simulink model "gm_commhdlQPSKTxRx"  (R2025b)
settings: Solver=VariableStepAuto  StartTime=0.0  StopTime=10.0  RelTol=1e-3
PostLoadFcn:
  | hScopeConfig = get_param([gcs '/Receiver/QPSK Rx/Frequency and Time Synchronizer/Symbol Synchronizer/No HDL/QPSK Receiver Eye Diagram'],'ScopeConfiguration');
  | 
  | hScopeConfig.OpenAtSimulationStart = false;
  | hScopeConfig.Visible = false;
  | SamplesPerSymbol = 4;
  | %UpsamplesRx = 1;
  | clear hScopeConfig
InitFcn:
  | commhdlQPSKTxRxModelInit;
  | % Rate bridge: ADRV9002/Jupiter radio runs at 15.36 MHz = 2x the 7.68 MHz
  | % (4 samples/symbol @ Rsym=1.92 MHz) the QPSK Rx requires. The deployed
  | % Receiver must downsample the ADC stream by 2. UpsamplesRx=1 fed the QPSK
  | % Rx 8 sps (2x-upsampled) and broke symbol sync / the loopback bit check.
  | UpsamplesRx = 2;
  | UpsamplesTx = 1;
  | clear simTimingOffset;
StopFcn:
  | if exist('simTimingOffset','var')
  |   disp('Simulation completed');
  |   %QPSKTxRxVerification;
  | end
undefined symbols (not defined in the file or in its folder): Add, Config, Error, fsym, Ignore, randsrc, RandStream, Rsym, Shift
libraries: hdlsllib x64, dspsigops x19, simulink x19, dsphdlfiltering2 x3, dsphdlsigops2 x2, dsphdlmathfun2 x2, commdigbbndpm3 x2, commchan3 x1, commrflib2 x1
(part 2 of 9)

== system gm_commhdlQPSKTxRx/Transmitter/QPSK Tx/HDL Data Scrambler ==
  note: HDL Data Scrambler
      | Polynomial: x^7+x^4+1
      | Initial state: [1 0 1 1 1 0 1]
  dataIn : Inport
  startIn : Inport  Port=2
  endIn : Inport  Port=3
  validIn : Inport  Port=4
  BIT_XOR : Logic  Operator=XOR  IconShape=distinctive  AllPortsSameDT=off  OutDataTypeStr=boolean
  BIT_XOR2 : Logic  Operator=XOR  IconShape=distinctive  AllPortsSameDT=off  OutDataTypeStr=boolean
  Delay{,1,3..4} (4 alike) : Delay  DelayLength=1
  EnableScrambling : Constant  Value=true  SampleTime=-1
  Logical Operator : Logic  IconShape=distinctive  AllPortsSameDT=off  OutDataTypeStr=boolean
  Switch : Switch  Criteria=u2 > Threshold  SaturateOnIntegerOverflow=off  InputSameDT=off
  Unit Delay Enabled Resettable Synchronous{,2..3,5,7} (5 alike) : hdlsllib/Discrete/Unit Delay Enabled Resettable Synchronous  InitialCondition=1  SampleTime=-1
  Unit Delay Enabled Resettable Synchronous1 : hdlsllib/Discrete/Unit Delay Enabled Resettable Synchronous  InitialCondition=0  SampleTime=-1
  Unit Delay Enabled Resettable Synchronous4 : hdlsllib/Discrete/Unit Delay Enabled Resettable Synchronous  InitialCondition=0  SampleTime=-1
  Unit Delay Enabled Resettable Synchronous6 : hdlsllib/Discrete/Unit Delay Enabled Resettable Synchronous  InitialCondition=0.0  SampleTime=-1
  dataOut : Outport  InitialOutput=0
  validOut : Outport  Port=2  InitialOutput=0
  wires:
  BIT_XOR2/1 -> Switch/1
  EnableScrambling/1 -> Switch/2
  Switch/1 -> Delay3/1
  Unit Delay Enabled Resettable Synchronous7/1 -> BIT_XOR/1
  Unit Delay Enabled Resettable Synchronous6/1 -> Unit Delay Enabled Resettable Synchronous7/1
  Unit Delay Enabled Resettable Synchronous5/1 -> Unit Delay Enabled Resettable Synchronous6/1
  Unit Delay Enabled Resettable Synchronous3/1 -> Unit Delay Enabled Resettable Synchronous5/1, BIT_XOR/2
  Unit Delay Enabled Resettable Synchronous/1 -> Unit Delay Enabled Resettable Synchronous1/1
  Unit Delay Enabled Resettable Synchronous2/1 -> Unit Delay Enabled Resettable Synchronous3/1
  Unit Delay Enabled Resettable Synchronous1/1 -> Unit Delay Enabled Resettable Synchronous2/1
  BIT_XOR/1 -> Logical Operator/2, Unit Delay Enabled Resettable Synchronous/1
  validIn/1 -> Delay1/1
  dataIn/1 -> Delay/1
  startIn/1 -> Unit Delay Enabled Resettable Synchronous7/3, Unit Delay Enabled Resettable Synchronous3/3, Unit Delay Enabled Resettable Synchronous2/3, Unit Delay Enabled Resettable Synchronous/3, Unit Delay Enabled Resettable Synchronous1/3, Unit Delay Enabled Resettable Synchronous5/3, Unit Delay Enabled Resettable Synchronous6/3, Unit Delay Enabled Resettable Synchronous4/2, Unit Delay Enabled Resettable Synchronous4/1
  Delay/1 -> BIT_XOR2/1, Switch/3
  Delay1/1 -> Unit Delay Enabled Resettable Synchronous7/2, Unit Delay Enabled Resettable Synchronous5/2, Unit Delay Enabled Resettable Synchronous3/2, Delay4/1, Unit Delay Enabled Resettable Synchronous/2, Unit Delay Enabled Resettable Synchronous1/2, Unit Delay Enabled Resettable Synchronous2/2, Unit Delay Enabled Resettable Synchronous6/2
  Unit Delay Enabled Resettable Synchronous4/1 -> Logical Operator/1
  Logical Operator/1 -> BIT_XOR2/2
  endIn/1 -> Unit Delay Enabled Resettable Synchronous4/3
  Delay3/1 -> dataOut/1
  Delay4/1 -> validOut/1

== system gm_commhdlQPSKTxRx/Transmitter/QPSK Tx/QPSK Modulator ==
  dataIn : Inport
  validIn : Inport  Port=2
  Compare To Constant : simulink/Logic and Bit Operations/Compare To Constant  relop===  const=0  OutDataTypeStr=boolean
  Compare To Constant1 : simulink/Logic and Bit Operations/Compare To Constant  relop===  const=1  OutDataTypeStr=boolean
  Delay{,1..5,11..12} (8 alike) : Delay  DelayLength=1
  HDL Counter : hdlsllib/Sources/HDL Counter  CountType=Count limited  CountInit=0  CountStep=1  CountMax=1  CountFromType=Initial value  CountFrom=0  CountResetPort=off  CountLoadPort=off  CountEnbPort=on  CountDirPort=off  CountHitOutputPort=off  CountDataType=Unsigned  CountWordLen=1  CountFracLen=0  CountSampTime=1
  Logical Operator : Logic  IconShape=distinctive  AllPortsSameDT=off  OutDataTypeStr=boolean
  Logical Operator1 : Logic  IconShape=distinctive  AllPortsSameDT=off  OutDataTypeStr=boolean
  Mux : Mux  Inputs=2
  Null : Constant  Value=complex(0,0)  OutDataTypeStr=fixdt(1,16,15)  SampleTime=1/(Rsym*4)
  QPSK Modulator Baseband : commdigbbndpm3/QPSK Modulator Baseband  InType=Bit  Enc=Gray  Ph=pi/4  outDtype=Fixed-point  outWordLen=16  outUDDataType=sfix(16)  outFracLenMode=User-defined  outFracLen=15  outDataTypeStr=fixdt(1,16,15)  outLastDataTypeStr=fixdt(1,16,15)
  Switch3 : Switch  Threshold=1  SaturateOnIntegerOverflow=off  InputSameDT=off
  Unit Delay Enabled Synchronous : hdlsllib/Discrete/Unit Delay Enabled Synchronous  InitialCondition=0.0  SampleTime=-1
  dataOut : Outport
  validOut : Outport  Port=2
  wires:
  Delay5/1 -> Delay12/1
  Delay4/1 -> QPSK Modulator Baseband/1
  Mux/1 -> Delay4/1
  Unit Delay Enabled Synchronous/1 -> Mux/1
  Logical Operator/1 -> Unit Delay Enabled Synchronous/2
  Delay12/1 -> Delay3/1, Switch3/2
  Delay11/1 -> Switch3/1
  Compare To Constant1/1 -> Logical Operator1/1
  Compare To Constant/1 -> Logical Operator/2
  Delay1/1 -> HDL Counter/1, Logical Operator/1, Logical Operator1/2
  Delay3/1 -> validOut/1
  Delay2/1 -> dataOut/1
  Delay/1 -> Unit Delay Enabled Synchronous/1, Mux/2
  Null/1 -> Switch3/3
  Switch3/1 -> Delay2/1
  Logical Operator1/1 -> Delay5/1
  QPSK Modulator Baseband/1 -> Delay11/1
  HDL Counter/1 -> Compare To Constant1/1, Compare To Constant/1
  validIn/1 -> Delay1/1
  dataIn/1 -> Delay/1

== system gm_commhdlQPSKTxRx/Transmitter/QPSK Tx/RRC Transmit Filter ==
  dataIn : Inport
  validIn : Inport  Port=2
  Data Type Conversion : DataTypeConversion  OutDataTypeStr=fixdt(1,17,16)  SaturateOnIntegerOverflow=off  RndMeth=Floor
  Data Type Conversion1 : DataTypeConversion  OutDataTypeStr=fixdt(1,16,14)  SaturateOnIntegerOverflow=off  RndMeth=Floor
  Delay1 : Delay  DelayLength=1
  Delay2 : Delay  DelayLength=1
  Delay3 : Delay  DelayLength=1
  RRC Filter : dsphdlfiltering2/Discrete FIR Filter  NumeratorSource=Property  Numerator=RRCCoef  NumeratorPrototype=[]  FilterStructure=Direct form systolic  SerializationOption=Minimum number of cycles between valid input samples  NumCycles=2  NumberOfMultipliers=2  SimulateUsing=Code generation  roundingMode=Floor  overflowMode=off  CoefficientsDataTypeStr=Inherit: Same word length as input  OutputDataTypeStr=Inherit: Same word length as input  ResetInputPort=off  HDLGlobalReset=off  CoeffMultiplier=Multiplier  UseMultForPow2Coeff=on  FrameInputSymmOptim=off
  Unit Delay Enabled Synchronous1 : hdlsllib/Discrete/Unit Delay Enabled Synchronous  InitialCondition=0  SampleTime=-1
  dataOut : Outport
  validOut : Outport  Port=2
  wires:
  Delay3/1 -> RRC Filter/1
  validIn/1 -> Unit Delay Enabled Synchronous1/1, Unit Delay Enabled Synchronous1/2
  Data Type Conversion1/1 -> Delay1/1
  Unit Delay Enabled Synchronous1/1 -> RRC Filter/2
  Data Type Conversion/1 -> Delay3/1
  Delay2/1 -> validOut/1
  Delay1/1 -> dataOut/1
  RRC Filter/2 -> Delay2/1
  RRC Filter/1 -> Data Type Conversion1/1
  dataIn/1 -> Data Type Conversion/1

== system gm_commhdlQPSKTxRx/Receiver/QPSK Rx/Automatic Gain Control/Error Detector ==
  dataIn : Inport  OutDataTypeStr=fixdt(1, 16, 14)  PortDimensions=1  SampleTime=1.30208333333333e-07
      settings: SignalType=complex
  Add1 : Sum  Inputs=+-  OutDataTypeStr=fixdt(1, 33, 28)
  Conj : Math  Operator=conj  OutDataTypeStr=fixdt(1, 16, 14)
  Delay{,1..3} (4 alike) : Delay
  Product : Product  OutDataTypeStr=fixdt(1, 32, 28)
  Ref : Constant  Value=Ref  OutDataTypeStr=fixdt(1, 16, 14)  SampleTime=-1
  err : Outport  SampleTime=1.30208333333333e-07
  wires:
  Delay3/1 -> err/1
  Add1/1 -> Delay3/1
  Delay2/1 -> Add1/2
  Ref/1 -> Add1/1
  Product/1 -> Delay2/1
  Delay/1 -> Product/2
  Delay1/1 -> Product/1
  Conj/1 -> Delay/1
  dataIn/1 -> Conj/1, Delay1/1

== system gm_commhdlQPSKTxRx/Receiver/QPSK Rx/Automatic Gain Control/Loop Filter ==
  err : Inport  OutDataTypeStr=fixdt(1, 33, 28)  PortDimensions=1  SampleTime=1.30208333333333e-07
      settings: SignalType=complex
  Add : Sum  Inputs=|++  OutDataTypeStr=fixdt(1, 33, 28)
  Delay1 : Delay  DelayLength=1
  Delay2 : Delay
  Delay3 : Delay
  Gain1 : Gain  Gain=LFG  OutDataTypeStr=fixdt(1, 33, 28)
      mask init:
      | Simulink.suppressDiagnostic(gcb, 'SimulinkFixedPoint:util:fxpParameterPrecisionLoss');
  gain : Outport  SampleTime=1.30208333333333e-07
  wires:
  Delay2/1 -> Add/1
  Add/1 -> Delay1/1
  Gain1/1 -> Delay2/1
  Delay3/1 -> Gain1/1
  Delay1/1 -> gain/1, Add/2
  err/1 -> Delay3/1

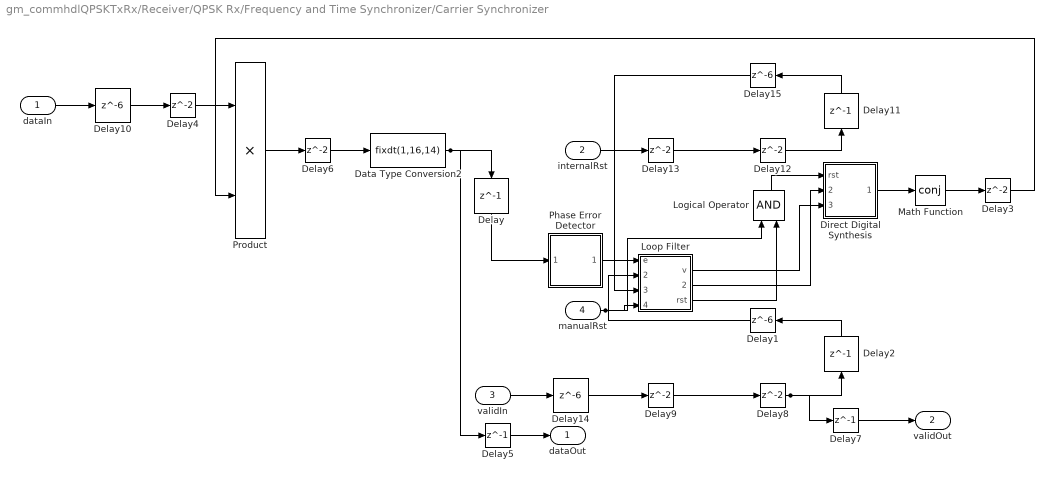
== system gm_commhdlQPSKTxRx/Receiver/QPSK Rx/Frequency and Time Synchronizer/Carrier Synchronizer ==
  dataIn : Inport  OutDataTypeStr=fixdt(1, 16, 14)  PortDimensions=1  SampleTime=1.30208333333333e-07
      settings: SignalType=complex
  internalRst : Inport  Port=2  OutDataTypeStr=boolean  PortDimensions=1  SampleTime=1.30208333333333e-07
  validIn : Inport  Port=3  OutDataTypeStr=boolean  PortDimensions=1  SampleTime=1.30208333333333e-07
  manualRst : Inport  Port=4  OutDataTypeStr=boolean  PortDimensions=1  SampleTime=1.30208333333333e-07
  Data Type Conversion2 : DataTypeConversion  OutDataTypeStr=fixdt(1,16,14)  SaturateOnIntegerOverflow=off  RndMeth=Floor
  Delay{,2,5,7,11} (5 alike) : Delay  DelayLength=1
  Delay{1,10,14..15} (4 alike) : Delay  DelayLength=6
  Delay{3..4,6,8..9,12..13} (7 alike) : Delay
  Direct Digital Synthesis : Subsystem
  Logical Operator : Logic  AllPortsSameDT=off  OutDataTypeStr=boolean
  Loop Filter : Subsystem
  Math Function : Math  Operator=conj  SignedPower=on  OutDataTypeStr=fixdt(1, 16, 14)  RndMeth=Zero
  Phase Error Detector : Subsystem
  Product : Product  OutDataTypeStr=fixdt(1, 32, 28)
  dataOut : Outport  SampleTime=1.30208333333333e-07
  validOut : Outport  Port=2  SampleTime=1.30208333333333e-07
  wires:
  Delay7/1 -> validOut/1
  Delay2/1 -> Delay1/1
  Logical Operator/1 -> Direct Digital Synthesis/1(rst)
  Direct Digital Synthesis/1(expOut) -> Math Function/1
  Delay1/1 -> Loop Filter/2(validIn)
  Loop Filter/3(rst) -> Logical Operator/2
  Delay9/1 -> Delay8/1
  Loop Filter/2(valid) -> Direct Digital Synthesis/2(validIn)
  Loop Filter/1(v) -> Direct Digital Synthesis/3(phaseInc)
  Math Function/1 -> Delay3/1
  Delay12/1 -> Delay11/1
  Delay13/1 -> Delay12/1
  Delay10/1 -> Delay4/1
  Delay3/1 -> Product/2
  Delay11/1 -> Delay15/1
  Data Type Conversion2/1 -> Delay5/1, Delay/1
  internalRst/1 -> Delay13/1
  Product/1 -> Delay6/1
  Delay5/1 -> dataOut/1
  Delay6/1 -> Data Type Conversion2/1
  Delay15/1 -> Loop Filter/3(internalRst)
  manualRst/1 -> Loop Filter/4(externalRst), Logical Operator/1
  Delay4/1 -> Product/1
  Delay14/1 -> Delay9/1
  Delay/1 -> Phase Error Detector/1(dataIn)
  Delay8/1 -> Delay7/1, Delay2/1
  dataIn/1 -> Delay10/1
  validIn/1 -> Delay14/1
  Phase Error Detector/1(PhaseError) -> Loop Filter/1(e)

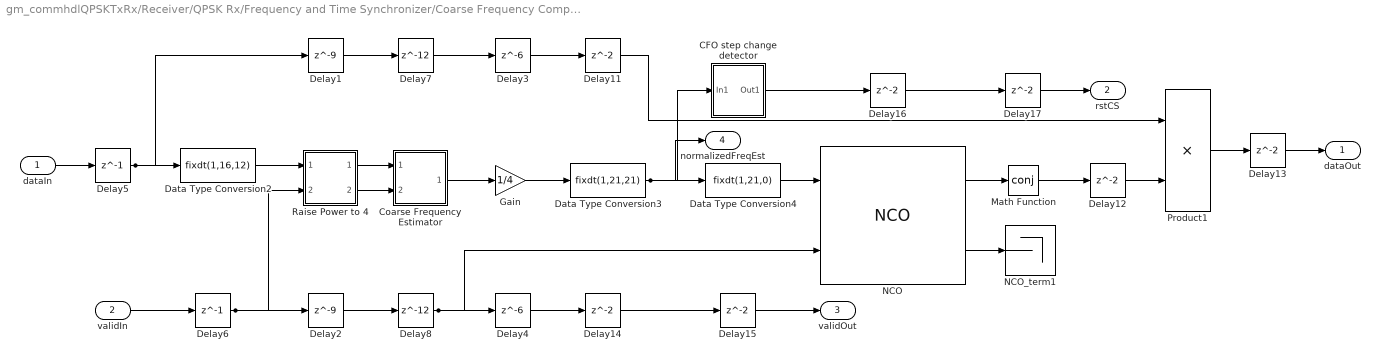
== system gm_commhdlQPSKTxRx/Receiver/QPSK Rx/Frequency and Time Synchronizer/Coarse Frequency Compensator ==
  dataIn : Inport  OutDataTypeStr=fixdt(1, 16, 14)  PortDimensions=1  SampleTime=1.30208333333333e-07
      settings: SignalType=complex
  validIn : Inport  Port=2  OutDataTypeStr=boolean  PortDimensions=1  SampleTime=1.30208333333333e-07
  CFO step change detector : Subsystem
  Coarse Frequency Estimator : Subsystem
  Data Type Conversion2 : DataTypeConversion  OutDataTypeStr=fixdt(1,16,12)  SaturateOnIntegerOverflow=off  RndMeth=Floor
  Data Type Conversion3 : DataTypeConversion  OutDataTypeStr=fixdt(1,21,21)  SaturateOnIntegerOverflow=off  RndMeth=Floor
  Data Type Conversion4 : DataTypeConversion  OutDataTypeStr=fixdt(1,21,0)  ConvertRealWorld=Stored Integer (SI)  SaturateOnIntegerOverflow=off  RndMeth=Floor
  Delay1 : Delay  DelayLength=9
  Delay{11..17} (7 alike) : Delay
  Delay2 : Delay  DelayLength=9
  Delay3 : Delay  DelayLength=6
  Delay4 : Delay  DelayLength=6
  Delay5 : Delay  DelayLength=1
  Delay6 : Delay  DelayLength=1
  Delay7 : Delay  DelayLength=12
  Delay8 : Delay  DelayLength=12
  Gain : Gain  Gain=1/4  ParamDataTypeStr=fixdt(0,2,2)  OutDataTypeStr=fixdt(1, 35, 34)
  Math Function : Math  Operator=conj  OutDataTypeStr=fixdt(1, 16, 14)
  NCO : dsphdlsigops2/NCO  PhaseIncrementSource=Input port  PhaseIncrement=100  PhaseOffsetSource=Property  PhaseOffset=0  DitherSource=None  NumDitherBits=4  SamplesPerFrame=1  LUTCompress=off  ResetAction=off  Waveform=Complex exponential  PhasePort=off  SimulateUsing=Code generation  AccumulatorWL=21  PhaseQuantization=on  NumQuantizerAccumulatorBits=14  OutputDataType=Binary point scaling  OutputWL=16  OutputFL=14
  NCO_term1 : Terminator
  Product1 : Product  OutDataTypeStr=fixdt(1, 16, 14)
  Raise Power to 4 : Subsystem
  dataOut : Outport  SampleTime=1.30208333333333e-07
  rstCS : Outport  Port=2  SampleTime=1.30208333333333e-07
  validOut : Outport  Port=3  SampleTime=1.30208333333333e-07
  normalizedFreqEst : Outport  Port=4  SampleTime=1.30208333333333e-07
  wires:
  Product1/1 -> Delay13/1
  Delay17/1 -> rstCS/1
  Delay16/1 -> Delay17/1
  CFO step change detector/1(Out1) -> Delay16/1
  Delay14/1 -> Delay15/1
  Delay13/1 -> dataOut/1
  Delay4/1 -> Delay14/1
  Gain/1 -> Data Type Conversion3/1
  dataIn/1 -> Delay5/1
  NCO/1 -> Math Function/1
  Delay5/1 -> Data Type Conversion2/1, Delay1/1
  Data Type Conversion2/1 -> Raise Power to 4/1(dataIn)
  Data Type Conversion4/1 -> NCO/1
  Delay6/1 -> Raise Power to 4/2(validIn), Delay2/1
  Delay11/1 -> Product1/1
  Delay7/1 -> Delay3/1
  Raise Power to 4/1(dataOut) -> Coarse Frequency Estimator/1(dataIn)
  Delay8/1 -> Delay4/1, NCO/2
  Delay12/1 -> Product1/2
  Math Function/1 -> Delay12/1
  validIn/1 -> Delay6/1
  Raise Power to 4/2(validOut) -> Coarse Frequency Estimator/2(validIn)
  Delay2/1 -> Delay8/1
  NCO/2 -> NCO_term1/1
  Delay15/1 -> validOut/1
  Delay1/1 -> Delay7/1
  Coarse Frequency Estimator/1(normFreqEst) -> Gain/1
  Data Type Conversion3/1 -> CFO step change detector/1(In1), normalizedFreqEst/1, Data Type Conversion4/1
  Delay3/1 -> Delay11/1

== system gm_commhdlQPSKTxRx/Receiver/QPSK Rx/Frequency and Time Synchronizer/Packet Controller ==
  dataIn : Inport  OutDataTypeStr=fixdt(1, 16, 14)  PortDimensions=1  SampleTime=1.30208333333333e-07
      settings: SignalType=complex
  syncPulse : Inport  Port=2  OutDataTypeStr=boolean  PortDimensions=1  SampleTime=1.30208333333333e-07
  validIn : Inport  Port=3  OutDataTypeStr=boolean  PortDimensions=1  SampleTime=1.30208333333333e-07
  Delay : Delay  DelayLength=4
  Delay1 : Delay  DelayLength=4
  Delay2 : Delay  DelayLength=4
  End Generator : Subsystem
  Logical Operator : Logic  IconShape=distinctive  AllPortsSameDT=off  OutDataTypeStr=boolean
  MATLAB Function : Subsystem
  sample discard controller : Subsystem
  dataOut : Outport  SampleTime=1.30208333333333e-07
  startOut : Outport  Port=2  SampleTime=1.30208333333333e-07
  endOut : Outport  Port=3  SampleTime=1.30208333333333e-07
  validOut : Outport  Port=4  SampleTime=1.30208333333333e-07
  wires:
  sample discard controller/1(dataOut) -> dataOut/1
  Logical Operator/1 -> End Generator/2(rst), Delay2/1
  sample discard controller/3(endOut) -> endOut/1
  End Generator/1(endOut) -> sample discard controller/4(endIn)
  Delay1/1 -> End Generator/1(validIn), sample discard controller/2(validIn)
  sample discard controller/4(validOut) -> validOut/1
  Delay/1 -> sample discard controller/1(dataIn)
  dataIn/1 -> Delay/1
  MATLAB Function/1(out) -> Logical Operator/2
  syncPulse/1 -> MATLAB Function/2(syncPulse)
  sample discard controller/2(startOut) -> startOut/1
  Delay2/1 -> sample discard controller/3(startIn)
  validIn/1 -> MATLAB Function/1(valid), Logical Operator/1, Delay1/1

== system gm_commhdlQPSKTxRx/Receiver/QPSK Rx/Frequency and Time Synchronizer/Phase Ambiguity Estimation and Correction ==
  dataIn : Inport  OutDataTypeStr=fixdt(1, 16, 14)  PortDimensions=1  SampleTime=1.30208333333333e-07
      settings: SignalType=complex
  syncPulseIn : Inport  Port=2  OutDataTypeStr=boolean  PortDimensions=1  SampleTime=1.30208333333333e-07
  validIn : Inport  Port=3  OutDataTypeStr=boolean  PortDimensions=1  SampleTime=1.30208333333333e-07
  Average Estimates : Subsystem
  Delay : Delay  DelayLength=32
  Delay1 : Delay  DelayLength=32
  Delay10 : Delay  DelayLength=15 + 7
  Delay11 : Delay  DelayLength=5
  Delay12 : Delay  DelayLength=5
  Delay13 : Delay  DelayLength=5
  Delay2 : Delay  DelayLength=32
  Delay3 : Delay  DelayLength=8
  Delay4 : Delay  DelayLength=8
  Delay5 : Delay  DelayLength=8
  Delay6 : Delay  DelayLength=1
  Delay7 : Delay  DelayLength=1
  Delay8 : Delay  DelayLength=1
  Delay9 : Delay  DelayLength=10
  Phase Ambiguity Corrector : Subsystem
  Phase Ambiguity Estimator : Subsystem
  dataOut : Outport  SampleTime=1.30208333333333e-07
  syncPulseOut : Outport  Port=2  SampleTime=1.30208333333333e-07
  validOut : Outport  Port=3  SampleTime=1.30208333333333e-07
  wires:
  Delay10/1 -> Delay9/1
  Delay9/1 -> syncPulseOut/1
  Phase Ambiguity Corrector/1(dataOut) -> dataOut/1
  Delay1/1 -> Delay11/1
  Delay7/1 -> Phase Ambiguity Corrector/3(validIn)
  Average Estimates/1(avgEst) -> Phase Ambiguity Corrector/2(estimate)
  Delay8/1 -> Phase Ambiguity Corrector/1(dataIn)
  dataIn/1 -> Delay5/1
  Delay11/1 -> Delay6/1
  Delay2/1 -> Phase Ambiguity Estimator/3(validIn), Delay12/1
  Phase Ambiguity Estimator/2(estOut) -> Average Estimates/2(estin)
  validIn/1 -> Delay4/1
  Delay5/1 -> Delay/1
  Delay12/1 -> Delay7/1
  Delay6/1 -> Delay10/1
  Delay4/1 -> Delay2/1
  Delay/1 -> Phase Ambiguity Estimator/1(dataIn), Delay13/1
  Phase Ambiguity Estimator/1(endOut) -> Average Estimates/1(endIn)
  Phase Ambiguity Corrector/2(validOut) -> validOut/1
  syncPulseIn/1 -> Phase Ambiguity Estimator/2(syncPulse), Delay3/1
  Phase Ambiguity Estimator/3(validOut) -> Average Estimates/3(validIn)
  Delay13/1 -> Delay8/1
  Delay3/1 -> Delay1/1

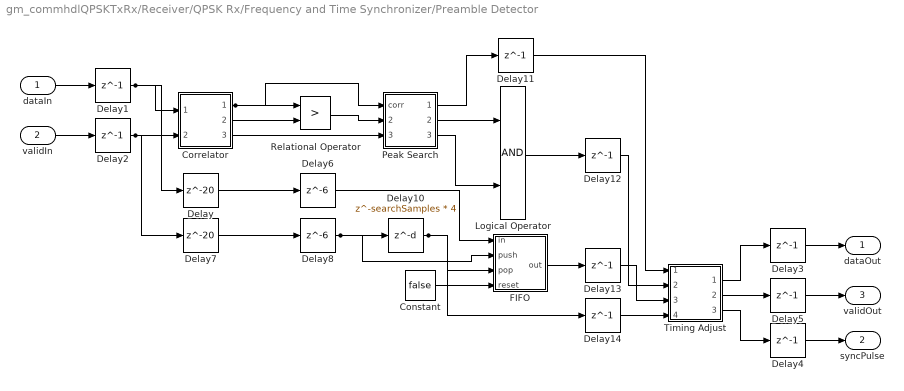
== system gm_commhdlQPSKTxRx/Receiver/QPSK Rx/Frequency and Time Synchronizer/Preamble Detector ==
  dataIn : Inport  OutDataTypeStr=fixdt(1, 16, 14)  PortDimensions=1  SampleTime=1.30208333333333e-07
      settings: SignalType=complex
  validIn : Inport  Port=2  OutDataTypeStr=boolean  PortDimensions=1  SampleTime=1.30208333333333e-07
  Constant : Constant  Value=false  OutDataTypeStr=boolean  SampleTime=-1
  Correlator : Subsystem
  Delay : Delay  DelayLength=20
  Delay{1..5,11..14} (9 alike) : Delay  DelayLength=1
  Delay10 : Delay  DelayLength=searchSamples * 4
  Delay6 : Delay  DelayLength=6
  Delay7 : Delay  DelayLength=20
  Delay8 : Delay  DelayLength=6
  FIFO : Subsystem  mask{fifoSize=double(1133), pushFullDiag=Error, popEmptyDiag=Error}
      mask prompts: fifoSize "FIFO size:"; pushFullDiag "Push full FIFO:"; popEmptyDiag "Pop empty FIFO:"
      mask TypeOptions pushFullDiag: Ignore | Warning | Error
      mask TypeOptions popEmptyDiag: Ignore | Warning | Error
  Logical Operator : Logic  AllPortsSameDT=off  OutDataTypeStr=boolean
  Peak Search : Subsystem  mask{samplesPerFrame=double(1133)}
      mask prompts: samplesPerFrame "Number of samples to search:"
      mask init:
      | samplesPerFrame = double(1133);
      | samplesPerFrame1x = double(1133);
      | searchDuration = double(1133);
  Relational Operator : RelationalOperator  Operator=>  OutDataTypeStr=boolean  InputSameDT=off
  Timing Adjust : Subsystem
  dataOut : Outport  SampleTime=1.30208333333333e-07
  syncPulse : Outport  Port=2  SampleTime=1.30208333333333e-07
  validOut : Outport  Port=3  SampleTime=1.30208333333333e-07
  wires:
  Delay4/1 -> syncPulse/1
  Timing Adjust/3(SyncPulse) -> Delay4/1
  Timing Adjust/2(validOut) -> Delay5/1
  Timing Adjust/1(dataOut) -> Delay3/1
  Delay14/1 -> Timing Adjust/4(validIn)
  Delay11/1 -> Timing Adjust/1(timingOffset)
  Delay10/1 -> FIFO/3(pop), Delay14/1
  Delay3/1 -> dataOut/1
  dataIn/1 -> Delay1/1
  Delay7/1 -> Delay8/1
  Constant/1 -> FIFO/4(reset)
  Delay6/1 -> FIFO/1(in)
  FIFO/1(out) -> Delay13/1
  Relational Operator/1 -> Peak Search/2(thresholdExceeded)
  Delay1/1 -> Correlator/1(dataIn), Delay/1
  Delay5/1 -> validOut/1
  Delay2/1 -> Correlator/2(validIn), Delay7/1
  Correlator/2(threshold) -> Relational Operator/2
  Correlator/3(validOut) -> Peak Search/3(validIn)
  Delay13/1 -> Timing Adjust/3(dataIn)
  validIn/1 -> Delay2/1
  Correlator/1(dataOut) -> Relational Operator/1, Peak Search/1(corr)
  Peak Search/1(timingOffset) -> Delay11/1
  Delay12/1 -> Timing Adjust/2(timingOffsetValid)
  Logical Operator/1 -> Delay12/1
  Peak Search/3(success) -> Logical Operator/2
  Delay/1 -> Delay6/1
  Peak Search/2(done) -> Logical Operator/1
  Delay8/1 -> Delay10/1, FIFO/2(push)

== system gm_commhdlQPSKTxRx/Receiver/QPSK Rx/Frequency and Time Synchronizer/Symbol Synchronizer ==
  dataIn : Inport  OutDataTypeStr=fixdt(1, 16, 12)  PortDimensions=1  SampleTime=1.30208333333333e-07
      settings: SignalType=complex
  validIn : Inport  Port=2  OutDataTypeStr=boolean  PortDimensions=1  SampleTime=1.30208333333333e-07
  Data Type Conversion4 : DataTypeConversion  OutDataTypeStr=fixdt(1,16,14)  SaturateOnIntegerOverflow=off  RndMeth=Floor
  Delay{1..4,6,8..9} (7 alike) : Delay  DelayLength=1
  Delay5 : Delay  DelayLength=12
  Delay7 : Delay  DelayLength=12
  Gardner TED : Subsystem
  Integer Delay{1..4} (4 alike) : Delay  DelayLength=1
  Interpolation Control : Subsystem
  Interpolation Filter : Subsystem
  Loop Filter : Subsystem
  Rate Handle : Subsystem
  dataOut : Outport  SampleTime=1.30208333333333e-07
  validOut : Outport  Port=2  SampleTime=1.30208333333333e-07
  wires:
  Rate Handle/2(validOut) -> validOut/1
  Rate Handle/1(dataOut) -> dataOut/1
  Delay6/1 -> Rate Handle/3(validIn)
  Delay2/1 -> Rate Handle/2(strobe)
  Data Type Conversion4/1 -> Rate Handle/1(dataIn)
  Delay1/1 -> Data Type Conversion4/1
  Integer Delay2/1 -> Delay7/1
  Delay5/1 -> Delay2/1, Delay9/1
  Interpolation Filter/1(interpolant) -> Delay1/1, Delay8/1
  Integer Delay3/1 -> Delay5/1
  dataIn/1 -> Integer Delay1/1
  Interpolation Control/1(mu) -> Integer Delay4/1
  Interpolation Control/2(Underflow) -> Integer Delay3/1
  Delay4/1 -> Interpolation Control/1(Delta)
  Delay7/1 -> Delay6/1
  Delay8/1 -> Gardner TED/1(data)
  validIn/1 -> Integer Delay2/1
  Loop Filter/1(v) -> Delay4/1
  Delay3/1 -> Loop Filter/1(e)
  Integer Delay4/1 -> Interpolation Filter/2(mu)
  Delay9/1 -> Gardner TED/2(strobe)
  Gardner TED/1(e) -> Delay3/1
  Integer Delay1/1 -> Interpolation Filter/1(In)

== system gm_commhdlQPSKTxRx/Receiver/QPSK Rx/QPSK Demodulator/Serializer ==
  u : Inport  OutDataTypeStr=boolean  PortDimensions=[2]  SampleTime=1.30208333333333e-07
  In2 : Inport  Port=2  OutDataTypeStr=boolean  PortDimensions=1  SampleTime=1.30208333333333e-07
  Delay1 : Delay  DelayLength=double(1)  InitialCondition=0  SampleTime=1.30208333333333e-07
  Delay4 : Delay  DelayLength=double(1)  InitialCondition=0  SampleTime=1.30208333333333e-07
  HDL Counter : hdlsllib/Sources/HDL Counter  CountType=Count limited  CountInit=0  CountStep=1  CountMax=1  CountFromType=Initial value  CountFrom=0  CountResetPort=off  CountLoadPort=off  CountEnbPort=on  CountDirPort=off  CountHitOutputPort=off  CountDataType=Unsigned  CountWordLen=1  CountFracLen=0  CountSampTime=1
  Logical Operator : Logic  Operator=OR  AllPortsSameDT=off  OutDataTypeStr=boolean  SampleTime=1.30208333333333e-07
  Multiport Switch : MultiPortSwitch  DataPortOrder=Zero-based contiguous  Inputs=2  DiagnosticForDefault=None  zeroidx=on  SampleTime=1.30208333333333e-07  SaturateOnIntegerOverflow=off  InputSameDT=off
  Unit Delay Enabled Synchronous : hdlsllib/Discrete/Unit Delay Enabled Synchronous  InitialCondition=double(0)  SampleTime=-1
  t : Demux  Outputs=2
  Out1 : Outport  SampleTime=1.30208333333333e-07
  Out2 : Outport  Port=2  SampleTime=1.30208333333333e-07
  wires:
  t/2 -> Multiport Switch/3
  HDL Counter/1 -> Multiport Switch/1
  Unit Delay Enabled Synchronous/1 -> t/1
  Logical Operator/1 -> HDL Counter/1, Out2/1
  Multiport Switch/1 -> Out1/1
  t/1 -> Multiport Switch/2
  u/1 -> Unit Delay Enabled Synchronous/1
  Delay4/1 -> Logical Operator/2
  Delay1/1 -> Delay4/1, Logical Operator/1
  In2/1 -> Delay1/1, Unit Delay Enabled Synchronous/2

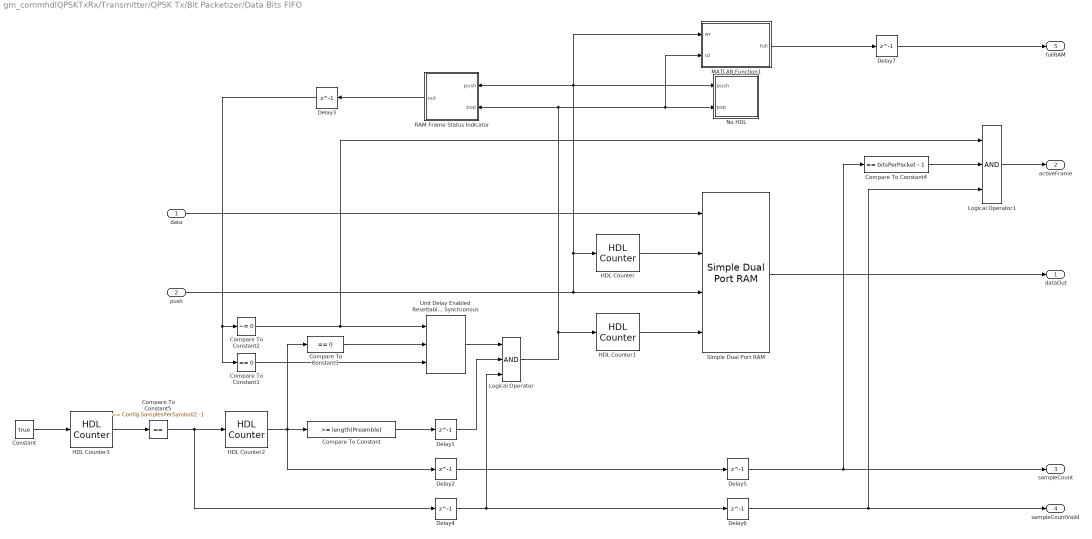
== system gm_commhdlQPSKTxRx/Transmitter/QPSK Tx/Bit Packetizer/Data Bits FIFO ==
  data : Inport
  push : Inport  Port=2
  Compare To Constant : simulink/Logic and Bit Operations/Compare To Constant  relop=>=  const=length(Preamble)  OutDataTypeStr=boolean
  Compare To Constant1 : simulink/Logic and Bit Operations/Compare To Constant  relop===  const=0  OutDataTypeStr=boolean
  Compare To Constant2 : simulink/Logic and Bit Operations/Compare To Constant  relop=~=  const=0  OutDataTypeStr=boolean
  Compare To Constant3 : simulink/Logic and Bit Operations/Compare To Constant  relop===  const=0  OutDataTypeStr=boolean
  Compare To Constant4 : simulink/Logic and Bit Operations/Compare To Constant  relop===  const=bitsPerPacket - 1  OutDataTypeStr=boolean
  Compare To Constant5 : hdlsllib/Logic and Bit Operations/Compare To Constant  relop===  const=Config.SamplesPerSymbol/2 -1  OutDataTypeStr=boolean
  Constant : Constant  Value=true  SampleTime=1/(Rsym*4)
  Delay{1..7} (7 alike) : Delay  DelayLength=1
  HDL Counter : hdlsllib/Sources/HDL Counter  CountType=Count limited  CountInit=0  CountStep=1  CountMax=dataBitsPerPacket*2 - 1  CountFromType=Initial value  CountFrom=0  CountResetPort=off  CountLoadPort=off  CountEnbPort=on  CountDirPort=off  CountHitOutputPort=off  CountDataType=Unsigned  CountWordLen=nextpow2(dataBitsPerPacket*2 - 1)  CountFracLen=0  CountSampTime=1
  HDL Counter1 : hdlsllib/Sources/HDL Counter  CountType=Count limited  CountInit=0  CountStep=1  CountMax=dataBitsPerPacket*2 - 1  CountFromType=Initial value  CountFrom=0  CountResetPort=off  CountLoadPort=off  CountEnbPort=on  CountDirPort=off  CountHitOutputPort=off  CountDataType=Unsigned  CountWordLen=nextpow2(dataBitsPerPacket*2 - 1)  CountFracLen=0  CountSampTime=1
  HDL Counter2 : hdlsllib/Sources/HDL Counter  CountType=Count limited  CountInit=0  CountStep=1  CountMax=bitsPerPacket - 1  CountFromType=Initial value  CountFrom=0  CountResetPort=off  CountLoadPort=off  CountEnbPort=on  CountDirPort=off  CountHitOutputPort=off  CountDataType=Unsigned  CountWordLen=nextpow2(bitsPerPacket)  CountFracLen=0  CountSampTime=1
  HDL Counter3 : hdlsllib/Sources/HDL Counter  CountType=Count limited  CountInit=0  CountStep=1  CountMax=Config.SamplesPerSymbol/2 -1  CountFromType=Initial value  CountFrom=0  CountResetPort=off  CountLoadPort=off  CountEnbPort=on  CountDirPort=off  CountHitOutputPort=off  CountDataType=Unsigned  CountWordLen=nextpow2(Config.SamplesPerSymbol/2)  CountFracLen=0  CountSampTime=1
  Logical Operator : Logic  Inputs=3  AllPortsSameDT=off  OutDataTypeStr=boolean
  Logical Operator1 : Logic  Inputs=3  AllPortsSameDT=off  OutDataTypeStr=boolean
  MATLAB Function1 : MATLAB Function  TreatAsAtomicUnit=on
  No HDL : Subsystem
  RAM Frame Status Indicator : MATLAB Function  TreatAsAtomicUnit=on
  Simple Dual Port RAM : hdlsllib/HDL RAMs/Simple Dual Port RAM  ram_size=nextpow2(dataBitsPerPacket*2 - 1)
  Unit Delay Enabled Resettable Synchronous : hdlsllib/Discrete/Unit Delay Enabled Resettable Synchronous  InitialCondition=0.0  SampleTime=-1
  dataOut : Outport
  activeFrame : Outport  Port=2
  sampleCount : Outport  Port=3
  sampleCountValid : Outport  Port=4
  fullRAM : Outport  Port=5
  wires:
  Compare To Constant5/1 -> Delay4/1, HDL Counter2/1
  HDL Counter3/1 -> Compare To Constant5/1
  Delay7/1 -> fullRAM/1
  MATLAB Function1/1(full) -> Delay7/1
  push/1 -> Simple Dual Port RAM/3, HDL Counter/1, No HDL/1(push), RAM Frame Status Indicator/1(push), MATLAB Function1/1(wr)
  Logical Operator/1 -> HDL Counter1/1, No HDL/2(pop), MATLAB Function1/2(rd), RAM Frame Status Indicator/2(pop)
  Logical Operator1/1 -> activeFrame/1
  Compare To Constant4/1 -> Logical Operator1/2
  Unit Delay Enabled Resettable Synchronous/1 -> Logical Operator/1
  Delay6/1 -> sampleCountValid/1, Logical Operator1/3
  Delay5/1 -> sampleCount/1, Compare To Constant4/1
  Delay4/1 -> Delay6/1, Logical Operator/3
  Simple Dual Port RAM/1 -> dataOut/1
  Delay3/1 -> Compare To Constant1/1, Compare To Constant2/1
  Delay2/1 -> Delay5/1
  Delay1/1 -> Logical Operator/2
  Compare To Constant/1 -> Delay1/1
  Compare To Constant3/1 -> Unit Delay Enabled Resettable Synchronous/2
  Compare To Constant2/1 -> Unit Delay Enabled Resettable Synchronous/1, Logical Operator1/1
  RAM Frame Status Indicator/1(out) -> Delay3/1
  Compare To Constant1/1 -> Unit Delay Enabled Resettable Synchronous/3
  HDL Counter2/1 -> Compare To Constant3/1, Delay2/1, Compare To Constant/1
  Constant/1 -> HDL Counter3/1
  data/1 -> Simple Dual Port RAM/1
  HDL Counter/1 -> Simple Dual Port RAM/2
  HDL Counter1/1 -> Simple Dual Port RAM/4

== system gm_commhdlQPSKTxRx/Transmitter/QPSK Tx/Bit Packetizer/Preamble Bits Generator ==
  activeFrame : Inport
  sampleCount : Inport  Port=2
  sampleCountValid : Inport  Port=3
  Compare To Constant2 : hdlsllib/Logic and Bit Operations/Compare To Constant  relop===  const=bitsPerPacket - 1  OutDataTypeStr=boolean
  Logical Operator3 : Logic  AllPortsSameDT=off  OutDataTypeStr=boolean
  Preamble Bits Store : Subsystem
  Unit Delay Enabled Synchronous : hdlsllib/Discrete/Unit Delay Enabled Synchronous  InitialCondition=0.0  SampleTime=-1
  preambleBits : Outport
  wires:
  activeFrame/1 -> Unit Delay Enabled Synchronous/1
  sampleCountValid/1 -> Logical Operator3/2
  Unit Delay Enabled Synchronous/1 -> Preamble Bits Store/1(actualPreamble)
  Compare To Constant2/1 -> Logical Operator3/1
  Preamble Bits Store/1(preamble) -> preambleBits/1
  Logical Operator3/1 -> Unit Delay Enabled Synchronous/2
  sampleCount/1 -> Preamble Bits Store/2(sampleCount), Compare To Constant2/1

== system gm_commhdlQPSKTxRx/Receiver/QPSK Rx/Frequency and Time Synchronizer/Carrier Synchronizer/Direct Digital Synthesis ==
  rst : Inport  OutDataTypeStr=boolean  PortDimensions=1  SampleTime=1.30208333333333e-07
  validIn : Inport  Port=2  OutDataTypeStr=boolean  PortDimensions=1  SampleTime=1.30208333333333e-07
  phaseInc : Inport  Port=3  OutDataTypeStr=fixdt(1, 40, 39)  PortDimensions=1  SampleTime=1.30208333333333e-07
  Data Type Conversion : DataTypeConversion  OutDataTypeStr=fixdt(1,21,21)  SaturateOnIntegerOverflow=off  RndMeth=Floor
  Data Type Conversion1 : DataTypeConversion  OutDataTypeStr=fixdt(1,21,0)  ConvertRealWorld=Stored Integer (SI)  SaturateOnIntegerOverflow=off  RndMeth=Floor
  Delay : Delay  DelayLength=1
  NCO : dsphdlsigops2/NCO  PhaseIncrementSource=Input port  PhaseIncrement=0  PhaseOffsetSource=Property  PhaseOffset=0  DitherSource=Property  NumDitherBits=11  SamplesPerFrame=1  LUTCompress=off  ResetAction=on  Waveform=Complex exponential  PhasePort=off  SimulateUsing=Code generation  AccumulatorWL=21  PhaseQuantization=on  NumQuantizerAccumulatorBits=14  OutputDataType=Binary point scaling  OutputWL=16  OutputFL=14
  NCO_term1 : Terminator
  expOut : Outport  SampleTime=1.30208333333333e-07
  wires:
  NCO/1 -> expOut/1
  rst/1 -> NCO/2
  NCO/2 -> NCO_term1/1
  Data Type Conversion1/1 -> NCO/1
  validIn/1 -> NCO/3
  Data Type Conversion/1 -> Data Type Conversion1/1
  Delay/1 -> Data Type Conversion/1
  phaseInc/1 -> Delay/1

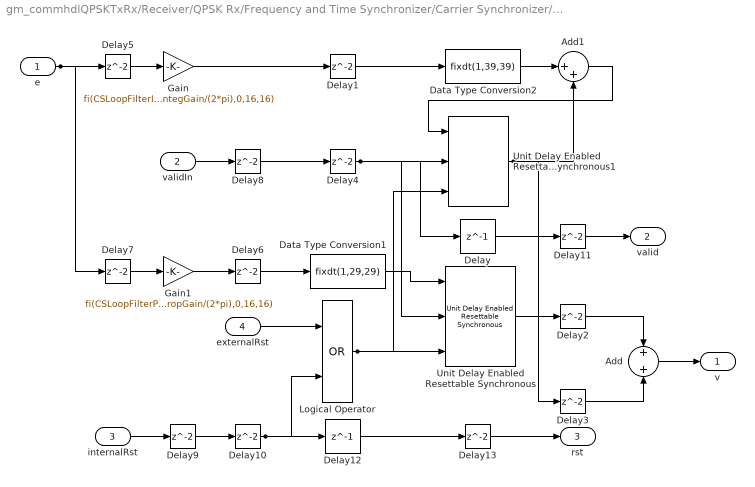
== system gm_commhdlQPSKTxRx/Receiver/QPSK Rx/Frequency and Time Synchronizer/Carrier Synchronizer/Loop Filter ==
  e : Inport  OutDataTypeStr=fixdt(1, 13, 10)  PortDimensions=1  SampleTime=1.30208333333333e-07
  validIn : Inport  Port=2  OutDataTypeStr=boolean  PortDimensions=1  SampleTime=1.30208333333333e-07
  internalRst : Inport  Port=3  OutDataTypeStr=boolean  PortDimensions=1  SampleTime=1.30208333333333e-07
  externalRst : Inport  Port=4  OutDataTypeStr=boolean  PortDimensions=1  SampleTime=1.30208333333333e-07
  Add : Sum  Inputs=+|+  OutDataTypeStr=fixdt(1, 40, 39)
  Add1 : Sum  Inputs=|++  OutDataTypeStr=fixdt(1, 39, 39)
  Data Type Conversion1 : DataTypeConversion  OutDataTypeStr=fixdt(1,29,29)  SaturateOnIntegerOverflow=off  RndMeth=Floor
  Data Type Conversion2 : DataTypeConversion  OutDataTypeStr=fixdt(1,39,39)  SaturateOnIntegerOverflow=off  RndMeth=Floor
  Delay : Delay  DelayLength=1
  Delay{1..11,13} (12 alike) : Delay
  Delay12 : Delay  DelayLength=1
  Gain : Gain  Gain=fi(CSLoopFilterIntegGain/(2*pi),0,16,16)  ParamDataTypeStr=Inherit: Inherit from 'Gain'  OutDataTypeStr=fixdt(1, 29, 26)
  Gain1 : Gain  Gain=fi(CSLoopFilterPropGain/(2*pi),0,16,16)  ParamDataTypeStr=Inherit: Inherit from 'Gain'  OutDataTypeStr=fixdt(1, 29, 26)
  Logical Operator : Logic  Operator=OR  AllPortsSameDT=off  OutDataTypeStr=boolean
  Unit Delay Enabled Resettable Synchronous : hdlsllib/Discrete/Unit Delay Enabled Resettable Synchronous  InitialCondition=0.0  SampleTime=-1
  Unit Delay Enabled Resettable Synchronous1 : hdlsllib/Discrete/Unit Delay Enabled Resettable Synchronous  InitialCondition=0.0  SampleTime=-1
  v : Outport  SampleTime=1.30208333333333e-07
  valid : Outport  Port=2  SampleTime=1.30208333333333e-07
  rst : Outport  Port=3  SampleTime=1.30208333333333e-07
  wires:
  Add/1 -> v/1
  Delay3/1 -> Add/2
  Delay11/1 -> valid/1
  Delay13/1 -> rst/1
  Unit Delay Enabled Resettable Synchronous/1 -> Delay2/1
  Add1/1 -> Unit Delay Enabled Resettable Synchronous1/1
  Unit Delay Enabled Resettable Synchronous1/1 -> Delay3/1, Add1/2
  Logical Operator/1 -> Unit Delay Enabled Resettable Synchronous/3, Unit Delay Enabled Resettable Synchronous1/3
  Data Type Conversion1/1 -> Unit Delay Enabled Resettable Synchronous/1
  Delay4/1 -> Delay/1, Unit Delay Enabled Resettable Synchronous1/2, Unit Delay Enabled Resettable Synchronous/2
  Delay2/1 -> Add/1
  e/1 -> Delay5/1, Delay7/1
  Delay5/1 -> Gain/1
  Delay12/1 -> Delay13/1
  Delay10/1 -> Delay12/1, Logical Operator/2
  Delay7/1 -> Gain1/1
  Delay6/1 -> Data Type Conversion1/1
  Delay/1 -> Delay11/1
  Data Type Conversion2/1 -> Add1/1
  externalRst/1 -> Logical Operator/1
  internalRst/1 -> Delay9/1
  validIn/1 -> Delay8/1
  Gain1/1 -> Delay6/1
  Gain/1 -> Delay1/1
  Delay9/1 -> Delay10/1
  Delay8/1 -> Delay4/1
  Delay1/1 -> Data Type Conversion2/1

== system gm_commhdlQPSKTxRx/Receiver/QPSK Rx/Frequency and Time Synchronizer/Carrier Synchronizer/Phase Error Detector ==
  dataIn : Inport  OutDataTypeStr=fixdt(1, 16, 14)  PortDimensions=1  SampleTime=1.30208333333333e-07
      settings: SignalType=complex
  Add : Sum  Inputs=+|-  OutDataTypeStr=fixdt(1, 19, 14)
  Compare To Constant : simulink/Logic and Bit Operations/Compare To Constant  relop=>=  const=0  OutDataTypeStr=boolean
  Compare To Constant1 : simulink/Logic and Bit Operations/Compare To Constant  relop=>=  const=0  OutDataTypeStr=boolean
  Complex to Real-Imag : ComplexToRealImag
  Constant : Constant  OutDataTypeStr=fixdt(1,2,0)  SampleTime=1/(Rsym*SamplesPerSymbol)
  Constant1 : Constant  Value=-1  OutDataTypeStr=fixdt(1,2,0)  SampleTime=1/(Rsym*SamplesPerSymbol)
  Constant2 : Constant  OutDataTypeStr=fixdt(1,2,0)  SampleTime=1/(Rsym*SamplesPerSymbol)
  Constant3 : Constant  Value=-1  OutDataTypeStr=fixdt(1,2,0)  SampleTime=1/(Rsym*SamplesPerSymbol)
  Data Type Conversion3 : DataTypeConversion  OutDataTypeStr=fixdt(1,10+3,10)  SaturateOnIntegerOverflow=off  RndMeth=Floor
  Delay{,1..6} (7 alike) : Delay
  Product : Product  OutDataTypeStr=fixdt(1, 18, 14)
  Product1 : Product  OutDataTypeStr=fixdt(1, 18, 14)
  Switch : Switch  Threshold=1  OutDataTypeStr=fixdt(1, 2, 0)  SaturateOnIntegerOverflow=off  InputSameDT=off
  Switch1 : Switch  Threshold=1  OutDataTypeStr=fixdt(1, 2, 0)  SaturateOnIntegerOverflow=off  InputSameDT=off
  PhaseError : Outport  SampleTime=1.30208333333333e-07
  wires:
  Delay6/1 -> Data Type Conversion3/1
  Add/1 -> Delay6/1
  Delay4/1 -> Add/1
  Delay3/1 -> Product1/2
  Delay2/1 -> Product1/1
  Constant1/1 -> Switch/3
  Complex to Real-Imag/1 -> Compare To Constant/1, Delay2/1
  Complex to Real-Imag/2 -> Compare To Constant1/1, Delay1/1
  Compare To Constant/1 -> Switch/2
  Constant2/1 -> Switch1/1
  Data Type Conversion3/1 -> PhaseError/1
  dataIn/1 -> Complex to Real-Imag/1
  Constant/1 -> Switch/1
  Delay1/1 -> Product/2
  Compare To Constant1/1 -> Switch1/2
  Constant3/1 -> Switch1/3
  Product/1 -> Delay4/1
  Switch/1 -> Delay/1
  Delay5/1 -> Add/2
  Product1/1 -> Delay5/1
  Switch1/1 -> Delay3/1
  Delay/1 -> Product/1

== system gm_commhdlQPSKTxRx/Receiver/QPSK Rx/Frequency and Time Synchronizer/Coarse Frequency Compensator/CFO step change detector ==
  note: fixed point precision loss warning supressed for this subsystem
  In1 : Inport  OutDataTypeStr=fixdt(1, 21, 21)  PortDimensions=1  SampleTime=1.30208333333333e-07
  Add : Sum  Inputs=+-  OutDataTypeStr=fixdt(1, 22, 21)
  Compare To Constant : simulink/Logic and Bit Operations/Compare To Constant  relop=>  const=fi(CFOChangeDetectThreshold,1,22,21)  OutDataTypeStr=boolean
  Compare To Constant1 : simulink/Logic and Bit Operations/Compare To Constant  relop=<  const=fi(-CFOChangeDetectThreshold,1,22,21)  OutDataTypeStr=boolean
  Delay : Delay  DelayLength=6
  Delay1 : Delay  DelayLength=1
  Logical Operator : Logic  Operator=OR  AllPortsSameDT=off  OutDataTypeStr=boolean
  Out1 : Outport  SampleTime=1.30208333333333e-07
  wires:
  Delay/1 -> Out1/1
  Compare To Constant1/1 -> Logical Operator/2
  Compare To Constant/1 -> Logical Operator/1
  Logical Operator/1 -> Delay/1
  Add/1 -> Compare To Constant/1, Compare To Constant1/1
  Delay1/1 -> Add/2
  In1/1 -> Delay1/1, Add/1

== system gm_commhdlQPSKTxRx/Receiver/QPSK Rx/Frequency and Time Synchronizer/Coarse Frequency Compensator/Coarse Frequency Estimator ==
  dataIn : Inport  OutDataTypeStr=fixdt(1, 16, 12)  PortDimensions=1  SampleTime=1.30208333333333e-07
      settings: SignalType=complex
  validIn : Inport  Port=2  OutDataTypeStr=boolean  PortDimensions=1  SampleTime=1.30208333333333e-07
  Delay{1,9..12} (5 alike) : Delay  DelayLength=1
  Delay{2..8} (7 alike) : Delay
  Extract Frequency : Subsystem
  Gain1 : Gain  Gain=1/integAvgLen  ParamDataTypeStr=fixdt(0,nextpow2(integAvgLen),nextpow2(integAvgLen))  OutDataTypeStr=fixdt(1, 32, 24)
  Integrator : Subsystem
  Math Function : Math  Operator=conj  OutDataTypeStr=fixdt(1, 16, 12)
  Product : Product  OutDataTypeStr=fixdt(1, 32, 24)
  Unit Delay Enabled Synchronous : hdlsllib/Discrete/Unit Delay Enabled Synchronous  InitialCondition=0.0  SampleTime=-1
  normFreqEst : Outport  SampleTime=1.30208333333333e-07
  wires:
  Extract Frequency/1(normFreqOut) -> normFreqEst/1
  Delay10/1 -> Extract Frequency/1(datain)
  Integrator/2(IntegValid) -> Delay11/1
  Delay5/1 -> Gain1/1
  Delay9/1 -> Delay6/1
  validIn/1 -> Delay9/1, Unit Delay Enabled Synchronous/2
  Integrator/1(IntegOut) -> Delay10/1
  Unit Delay Enabled Synchronous/1 -> Delay12/1
  Delay4/1 -> Integrator/2(validIn)
  Delay1/1 -> Delay7/1
  Delay2/1 -> Integrator/1(dataIn)
  Gain1/1 -> Delay2/1
  Delay12/1 -> Math Function/1
  Delay3/1 -> Delay4/1
  Delay11/1 -> Extract Frequency/2(validIn)
  Delay7/1 -> Product/1
  dataIn/1 -> Unit Delay Enabled Synchronous/1, Delay1/1
  Delay8/1 -> Product/2
  Delay6/1 -> Delay3/1
  Math Function/1 -> Delay8/1
  Product/1 -> Delay5/1

== system gm_commhdlQPSKTxRx/Receiver/QPSK Rx/Frequency and Time Synchronizer/Coarse Frequency Compensator/Raise Power to 4 ==
  dataIn : Inport  OutDataTypeStr=fixdt(1, 16, 12)  PortDimensions=1  SampleTime=1.30208333333333e-07
      settings: SignalType=complex
  validIn : Inport  Port=2  OutDataTypeStr=boolean  PortDimensions=1  SampleTime=1.30208333333333e-07
  Delay{1..8,11..12} (10 alike) : Delay
  Delay10 : Delay  DelayLength=1
  Delay9 : Delay  DelayLength=1
  Product1 : Product  OutDataTypeStr=fixdt(1, 16, 12)
  Product2 : Product  OutDataTypeStr=fixdt(1, 16, 12)
  dataOut : Outport  SampleTime=1.30208333333333e-07
  validOut : Outport  Port=2  SampleTime=1.30208333333333e-07
  wires:
  Delay11/1 -> dataOut/1
  Product2/1 -> Delay11/1
  Delay12/1 -> validOut/1
  dataIn/1 -> Delay3/1, Delay4/1
  validIn/1 -> Delay5/1
  Delay10/1 -> Delay8/1
  Delay9/1 -> Delay6/1, Delay7/1
  Delay6/1 -> Product2/1
  Delay5/1 -> Delay2/1
  Delay3/1 -> Product1/1
  Product1/1 -> Delay1/1
  Delay8/1 -> Delay12/1
  Delay2/1 -> Delay10/1
  Delay1/1 -> Delay9/1
  Delay4/1 -> Product1/2
  Delay7/1 -> Product2/2

== system gm_commhdlQPSKTxRx/Receiver/QPSK Rx/Frequency and Time Synchronizer/Packet Controller/End Generator ==
  validIn : Inport  OutDataTypeStr=boolean  PortDimensions=1  SampleTime=1.30208333333333e-07
  rst : Inport  Port=2  OutDataTypeStr=boolean  PortDimensions=1  SampleTime=1.30208333333333e-07
  Compare To Constant : simulink/Logic and Bit Operations/Compare To Constant  relop===  const=1120-1  OutDataTypeStr=boolean
  Delay6 : Delay  DelayLength=1
  HDL Counter : hdlsllib/Sources/HDL Counter  CountType=Count limited  CountInit=0  CountStep=1  CountMax=1120 -1  CountFromType=Initial value  CountFrom=0  CountResetPort=on  CountLoadPort=off  CountEnbPort=on  CountDirPort=off  CountHitOutputPort=off  CountDataType=Unsigned  CountWordLen=nextpow2(1120-1)  CountFracLen=0  CountSampTime=1
  Logical Operator1 : Logic  IconShape=distinctive  AllPortsSameDT=off  OutDataTypeStr=boolean
  endOut : Outport  SampleTime=1.30208333333333e-07
  wires:
  Logical Operator1/1 -> Delay6/1
  Compare To Constant/1 -> Logical Operator1/1
  Delay6/1 -> endOut/1
  HDL Counter/1 -> Compare To Constant/1
  validIn/1 -> HDL Counter/2, Logical Operator1/2
  rst/1 -> HDL Counter/1

== system gm_commhdlQPSKTxRx/Receiver/QPSK Rx/Frequency and Time Synchronizer/Packet Controller/MATLAB Function ==
  valid : Inport  OutDataTypeStr=boolean  PortDimensions=1  SampleTime=1.30208333333333e-07
  syncPulse : Inport  Port=2  OutDataTypeStr=boolean  PortDimensions=1  SampleTime=1.30208333333333e-07
  MATLAB Function : MATLAB Function  TreatAsAtomicUnit=on
  out : Outport  SampleTime=1.30208333333333e-07  VectorParamsAs1DForOutWhenUnconnected=off
  wires:
  MATLAB Function/1(out) -> out/1
  syncPulse/1 -> MATLAB Function/2(syncPulse)
  valid/1 -> MATLAB Function/1(valid)

== system gm_commhdlQPSKTxRx/Receiver/QPSK Rx/Frequency and Time Synchronizer/Packet Controller/sample discard controller ==
  dataIn : Inport  OutDataTypeStr=fixdt(1, 16, 14)  PortDimensions=1  SampleTime=1.30208333333333e-07
      settings: SignalType=complex
  validIn : Inport  Port=2  OutDataTypeStr=boolean  PortDimensions=1  SampleTime=1.30208333333333e-07
  startIn : Inport  Port=3  OutDataTypeStr=boolean  PortDimensions=1  SampleTime=1.30208333333333e-07
  endIn : Inport  Port=4  OutDataTypeStr=boolean  PortDimensions=1  SampleTime=1.30208333333333e-07
  sample discard controller : MATLAB Function  TreatAsAtomicUnit=on
  dataOut : Outport  SampleTime=1.30208333333333e-07  VectorParamsAs1DForOutWhenUnconnected=off
  startOut : Outport  Port=2  SampleTime=1.30208333333333e-07
  endOut : Outport  Port=3  SampleTime=1.30208333333333e-07
  validOut : Outport  Port=4  SampleTime=1.30208333333333e-07
  wires:
  sample discard controller/3(endOut) -> endOut/1
  sample discard controller/4(validOut) -> validOut/1
  sample discard controller/2(startOut) -> startOut/1
  endIn/1 -> sample discard controller/4(endIn)
  startIn/1 -> sample discard controller/3(startIn)
  sample discard controller/1(dataOut) -> dataOut/1
  validIn/1 -> sample discard controller/2(validIn)
  dataIn/1 -> sample discard controller/1(dataIn)

== system gm_commhdlQPSKTxRx/Receiver/QPSK Rx/Frequency and Time Synchronizer/Phase Ambiguity Estimation and Correction/Average Estimates ==
  endIn : Inport  OutDataTypeStr=boolean  PortDimensions=1  SampleTime=1.30208333333333e-07
  estin : Inport  Port=2  OutDataTypeStr=fixdt(1, 32, 29)  PortDimensions=1  SampleTime=1.30208333333333e-07
      settings: SignalType=complex
  validIn : Inport  Port=3  OutDataTypeStr=boolean  PortDimensions=1  SampleTime=1.30208333333333e-07
  Add : Sum  Inputs=++|  OutDataTypeStr=fixdt(1, 25, 13)
  Data Type Conversion : DataTypeConversion  OutDataTypeStr=fixdt(1,16+8,13)  SaturateOnIntegerOverflow=off  RndMeth=Floor
  Data Type Conversion1 : DataTypeConversion  OutDataTypeStr=fixdt(1,16+8,13)  SaturateOnIntegerOverflow=off  RndMeth=Floor
  Data Type Conversion2 : DataTypeConversion  OutDataTypeStr=fixdt(1,16,14)  SaturateOnIntegerOverflow=off  RndMeth=Floor
  Delay{,1..3} (4 alike) : Delay  DelayLength=1
  Divide by 8 : DataTypeConversion  OutDataTypeStr=fixdt(1,24,13+log2(8))  ConvertRealWorld=Stored Integer (SI)  SaturateOnIntegerOverflow=off  RndMeth=Floor
  Unit Delay Enabled Resettable Synchronous : hdlsllib/Discrete/Unit Delay Enabled Resettable Synchronous  InitialCondition=0.0  SampleTime=-1
  Unit Delay Enabled Synchronous : hdlsllib/Discrete/Unit Delay Enabled Synchronous  InitialCondition=0.0  SampleTime=-1
  avgEst : Outport  SampleTime=1.30208333333333e-07
  wires:
  endIn/1 -> Delay2/1
  Delay/1 -> Data Type Conversion/1
  validIn/1 -> Delay1/1
  estin/1 -> Delay/1
  Delay2/1 -> Delay3/1, Unit Delay Enabled Synchronous/2
  Delay1/1 -> Unit Delay Enabled Resettable Synchronous/2
  Data Type Conversion/1 -> Add/2
  Data Type Conversion2/1 -> avgEst/1
  Divide by 8/1 -> Unit Delay Enabled Synchronous/1
  Delay3/1 -> Unit Delay Enabled Resettable Synchronous/3
  Data Type Conversion1/1 -> Unit Delay Enabled Resettable Synchronous/1
  Unit Delay Enabled Resettable Synchronous/1 -> Divide by 8/1, Add/1
  Unit Delay Enabled Synchronous/1 -> Data Type Conversion2/1
  Add/1 -> Data Type Conversion1/1
